simulink model "simlwrkuka_kinematics"  (R2014a)
settings: Solver=ode1  StartTime=0.0  StopTime=7  FixedStep=0.001  MaxStep=0.00001  RelTol=1e-3
values from neighbouring files (symbols this model uses):
  qi = [pi/2;0;0;pi/2;0;pi/2;pi/6]    [initial.m]
settings Model: Creator=Admin  LastModifiedBy=faezeh

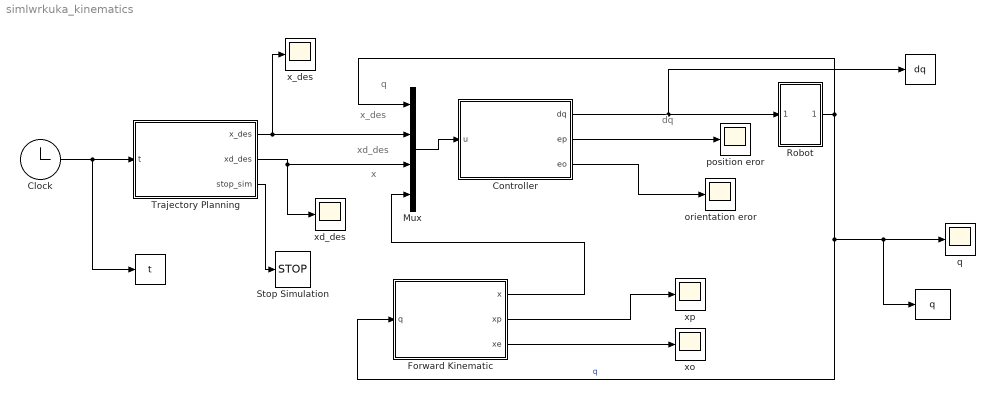
== system simlwrkuka_kinematics ==
  note: x
  note: dq
  note: q
  note: x_des
  note: xd_des
  " " : ToWorkspace  VariableName=q  SampleTime=-1
  "  " : ToWorkspace  VariableName=dq  SampleTime=-1
  " " : ToWorkspace  VariableName=t  SampleTime=-1
  Clock : Clock
  Controller : MATLAB Function  TreatAsAtomicUnit=on
  Forward Kinematic : MATLAB Function  TreatAsAtomicUnit=on
  Mux : Mux
  Robot : Subsystem
  Stop Simulation : Stop
  Trajectory Planning : MATLAB Function  TreatAsAtomicUnit=on
  orientation eror : Scope
  position eror : Scope
  q : Scope
      settings: SaveName=ScopeData2
  "x_des " : Scope
      settings: SaveName=ScopeData5
  "xd_des " : Scope
      settings: SaveName=ScopeData6
  xo : Scope
      settings: SaveName=ScopeData4
  xp : Scope
      settings: SaveName=ScopeData3
  wires:
  Clock/1 -> " "/1, Trajectory Planning/1(t)
  Trajectory Planning/3(stop_sim) -> Stop Simulation/1
  Mux/1 -> Controller/1(u)
  Controller/2(ep) -> position eror/1
  Trajectory Planning/1(x_des) -> "x_des "/1, Mux/2
  Trajectory Planning/2(xd_des) -> "xd_des "/1, Mux/3
  Controller/1(dq) -> "  "/1, Robot/1(In1)
  Robot/1(Out1) -> Forward Kinematic/1(q), " "/1, q/1, Mux/1  "q"
  Controller/3(eo) -> orientation eror/1
  Forward Kinematic/1(x) -> Mux/4
  Forward Kinematic/2(xp) -> xp/1
  Forward Kinematic/3(xe) -> xo/1

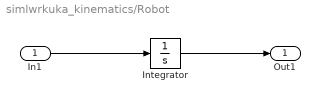
== system simlwrkuka_kinematics/Robot ==
  In1 : Inport
  Integrator : Integrator  InitialCondition=qi
  Out1 : Outport
  wires:
  Integrator/1 -> Out1/1
  In1/1 -> Integrator/1

== matlab function simlwrkuka_kinematics/Controller ==
  data: u input; dq output; ep output; eo output
function [dq,ep,eo] = command(u)
q1=u(1);q2=u(2);q3=u(3);q4=u(4);q5=u(5);q6=u(6);q7=u(7);
x_des=[u(8);u(9);u(10);u(11);u(12);u(13);u(14)];
xd_des=[u(15);u(16);u(17);u(18);u(19);u(20)];
x=[u(21);u(22);u(23);u(24);u(25);u(26);u(27)];
% J=[   (2*sin(q1)*sin(q2))/5 - (39*sin(q4)*(cos(q1)*sin(q3) + cos(q2)*cos(q3)*sin(q1)))/100 + (39*cos(q4)*sin(q1)*sin(q2))/100,                                                                                                                                                                                  -cos(q1)*((2*cos(q2))/5 + (39*cos(q2)*cos(q4))/100 + (39*cos(q3)*sin(q2)*sin(q4))/100),                                                     cos(q2)*((2*sin(q1)*sin(q2))/5 - (39*sin(q4)*(cos(q1)*sin(q3) + cos(q2)*cos(q3)*sin(q1)))/100 + (39*cos(q4)*sin(q1)*sin(q2))/100) - sin(q1)*sin(q2)*((2*cos(q2))/5 + (39*cos(q2)*cos(q4))/100 + (39*cos(q3)*sin(q2)*sin(q4))/100),                                                                 (cos(q1)*cos(q3) - cos(q2)*sin(q1)*sin(q3))*((39*cos(q2)*cos(q4))/100 + (39*cos(q3)*sin(q2)*sin(q4))/100) + sin(q2)*sin(q3)*((39*sin(q4)*(cos(q1)*sin(q3) + cos(q2)*cos(q3)*sin(q1)))/100 - (39*cos(q4)*sin(q1)*sin(q2))/100),                                                                         (sin(q4)*(cos(q1)*sin(q3) + cos(q2)*cos(q3)*sin(q1)) - cos(q4)*sin(q1)*sin(q2))*((39*cos(q2)*cos(q4))/100 + (39*cos(q3)*sin(q2)*sin(q4))/100) - ((39*sin(q4)*(cos(q1)*sin(q3) + cos(q2)*cos(q3)*sin(q1)))/100 - (39*cos(q4)*sin(q1)*sin(q2))/100)*(cos(q2)*cos(q4) + cos(q3)*sin(q2)*sin(q4)),                                                                                                                                             0,                                                                                                                                                                                                                                                 0
%  - (2*cos(q1)*sin(q2))/5 - (39*sin(q4)*(sin(q1)*sin(q3) - cos(q1)*cos(q2)*cos(q3)))/100 - (39*cos(q1)*cos(q4)*sin(q2))/100,                                                                                                                                                                                  -sin(q1)*((2*cos(q2))/5 + (39*cos(q2)*cos(q4))/100 + (39*cos(q3)*sin(q2)*sin(q4))/100),                                                     cos(q1)*sin(q2)*((2*cos(q2))/5 + (39*cos(q2)*cos(q4))/100 + (39*cos(q3)*sin(q2)*sin(q4))/100) - cos(q2)*((2*cos(q1)*sin(q2))/5 + (39*sin(q4)*(sin(q1)*sin(q3) - cos(q1)*cos(q2)*cos(q3)))/100 + (39*cos(q1)*cos(q4)*sin(q2))/100),                                                                 (cos(q3)*sin(q1) + cos(q1)*cos(q2)*sin(q3))*((39*cos(q2)*cos(q4))/100 + (39*cos(q3)*sin(q2)*sin(q4))/100) + sin(q2)*sin(q3)*((39*sin(q4)*(sin(q1)*sin(q3) - cos(q1)*cos(q2)*cos(q3)))/100 + (39*cos(q1)*cos(q4)*sin(q2))/100),                                                                         ((39*cos(q2)*cos(q4))/100 + (39*cos(q3)*sin(q2)*sin(q4))/100)*(sin(q4)*(sin(q1)*sin(q3) - cos(q1)*cos(q2)*cos(q3)) + cos(q1)*cos(q4)*sin(q2)) - (cos(q2)*cos(q4) + cos(q3)*sin(q2)*sin(q4))*((39*sin(q4)*(sin(q1)*sin(q3) - cos(q1)*cos(q2)*cos(q3)))/100 + (39*cos(q1)*cos(q4)*sin(q2))/100),                                                                                                                                             0,                                                                                                                                                                                                                                                 0
%                                                                                                                          0, - cos(q1)*((2*cos(q1)*sin(q2))/5 + (39*sin(q4)*(sin(q1)*sin(q3) - cos(q1)*cos(q2)*cos(q3)))/100 + (39*cos(q1)*cos(q4)*sin(q2))/100) - sin(q1)*((2*sin(q1)*sin(q2))/5 - (39*sin(q4)*(cos(q1)*sin(q3) + cos(q2)*cos(q3)*sin(q1)))/100 + (39*cos(q4)*sin(q1)*sin(q2))/100), cos(q1)*sin(q2)*((2*sin(q1)*sin(q2))/5 - (39*sin(q4)*(cos(q1)*sin(q3) + cos(q2)*cos(q3)*sin(q1)))/100 + (39*cos(q4)*sin(q1)*sin(q2))/100) - sin(q1)*sin(q2)*((2*cos(q1)*sin(q2))/5 + (39*sin(q4)*(sin(q1)*sin(q3) - cos(q1)*cos(q2)*cos(q3)))/100 + (39*cos(q1)*cos(q4)*sin(q2))/100), (cos(q1)*cos(q3) - cos(q2)*sin(q1)*sin(q3))*((39*sin(q4)*(sin(q1)*sin(q3) - cos(q1)*cos(q2)*cos(q3)))/100 + (39*cos(q1)*cos(q4)*sin(q2))/100) - ((39*sin(q4)*(cos(q1)*sin(q3) + cos(q2)*cos(q3)*sin(q1)))/100 - (39*cos(q4)*sin(q1)*sin(q2))/100)*(cos(q3)*sin(q1) + cos(q1)*cos(q2)*sin(q3)), (sin(q4)*(cos(q1)*sin(q3) + cos(q2)*cos(q3)*sin(q1)) - cos(q4)*sin(q1)*sin(q2))*((39*sin(q4)*(sin(q1)*sin(q3) - cos(q1)*cos(q2)*cos(q3)))/100 + (39*cos(q1)*cos(q4)*sin(q2))/100) - ((39*sin(q4)*(cos(q1)*sin(q3) + cos(q2)*cos(q3)*sin(q1)))/100 - (39*cos(q4)*sin(q1)*sin(q2))/100)*(sin(q4)*(sin(q1)*sin(q3) - cos(q1)*cos(q2)*cos(q3)) + cos(q1)*cos(q4)*sin(q2)),                                                                                                                                             0,                                                                                                                                                                                                                                                 0
%                                                                                                                          0,                                                                                                                                                                                                                                                                 sin(q1),                                                                                                                                                                                                                                                                      -cos(q1)*sin(q2),                                                                                                                                                                                                                                                   - cos(q3)*sin(q1) - cos(q1)*cos(q2)*sin(q3),                                                                                                                                                                                                                                                                                       - sin(q4)*(sin(q1)*sin(q3) - cos(q1)*cos(q2)*cos(q3)) - cos(q1)*cos(q4)*sin(q2), cos(q5)*(cos(q3)*sin(q1) + cos(q1)*cos(q2)*sin(q3)) - sin(q5)*(cos(q4)*(sin(q1)*sin(q3) - cos(q1)*cos(q2)*cos(q3)) - cos(q1)*sin(q2)*sin(q4)), sin(q6)*(cos(q5)*(cos(q4)*(sin(q1)*sin(q3) - cos(q1)*cos(q2)*cos(q3)) - cos(q1)*sin(q2)*sin(q4)) + sin(q5)*(cos(q3)*sin(q1) + cos(q1)*cos(q2)*sin(q3))) - cos(q6)*(sin(q4)*(sin(q1)*sin(q3) - cos(q1)*cos(q2)*cos(q3)) + cos(q1)*cos(q4)*sin(q2))
%                                                                                                                          0,                                                                                                                                                                                                                                                                -cos(q1),                                                                                                                                                                                                                                                                      -sin(q1)*sin(q2),                                                                                                                                                                                                                                                     cos(q1)*cos(q3) - cos(q2)*sin(q1)*sin(q3),                                                                                                                                                                                                                                                                                         sin(q4)*(cos(q1)*sin(q3) + cos(q2)*cos(q3)*sin(q1)) - cos(q4)*sin(q1)*sin(q2), sin(q5)*(cos(q4)*(cos(q1)*sin(q3) + cos(q2)*cos(q3)*sin(q1)) + sin(q1)*sin(q2)*sin(q4)) - cos(q5)*(cos(q1)*cos(q3) - cos(q2)*sin(q1)*sin(q3)), cos(q6)*(sin(q4)*(cos(q1)*sin(q3) + cos(q2)*cos(q3)*sin(q1)) - cos(q4)*sin(q1)*sin(q2)) - sin(q6)*(cos(q5)*(cos(q4)*(cos(q1)*sin(q3) + cos(q2)*cos(q3)*sin(q1)) + sin(q1)*sin(q2)*sin(q4)) + sin(q5)*(cos(q1)*cos(q3) - cos(q2)*sin(q1)*sin(q3)))
%                                                                                                                          1,                                                                                                                                                                                                                                                                       0,                                                                                                                                                                                                                                                                               cos(q2),                                                                                                                                                                                                                                                                              -sin(q2)*sin(q3),                                                                                                                                                                                                                                                                                                                             cos(q2)*cos(q4) + cos(q3)*sin(q2)*sin(q4),                                                                 cos(q5)*sin(q2)*sin(q3) - sin(q5)*(cos(q2)*sin(q4) - cos(q3)*cos(q4)*sin(q2)),                                                                                                     sin(q6)*(cos(q5)*(cos(q2)*sin(q4) - cos(q3)*cos(q4)*sin(q2)) + sin(q2)*sin(q3)*sin(q5)) + cos(q6)*(cos(q2)*cos(q4) + cos(q3)*sin(q2)*sin(q4))];
% T7=[ sin(q7)*(sin(q5)*(cos(q4)*(sin(q1)*sin(q3) - cos(q1)*cos(q2)*cos(q3)) - cos(q1)*sin(q2)*sin(q4)) - cos(q5)*(cos(q3)*sin(q1) + cos(q1)*cos(q2)*sin(q3))) - cos(q7)*(sin(q6)*(sin(q4)*(sin(q1)*sin(q3) - cos(q1)*cos(q2)*cos(q3)) + cos(q1)*cos(q4)*sin(q2)) + cos(q6)*(cos(q5)*(cos(q4)*(sin(q1)*sin(q3) - cos(q1)*cos(q2)*cos(q3)) - cos(q1)*sin(q2)*sin(q4)) + sin(q5)*(cos(q3)*sin(q1) + cos(q1)*cos(q2)*sin(q3)))),   sin(q7)*(sin(q6)*(sin(q4)*(sin(q1)*sin(q3) - cos(q1)*cos(q2)*cos(q3)) + cos(q1)*cos(q4)*sin(q2)) + cos(q6)*(cos(q5)*(cos(q4)*(sin(q1)*sin(q3) - cos(q1)*cos(q2)*cos(q3)) - cos(q1)*sin(q2)*sin(q4)) + sin(q5)*(cos(q3)*sin(q1) + cos(q1)*cos(q2)*sin(q3)))) + cos(q7)*(sin(q5)*(cos(q4)*(sin(q1)*sin(q3) - cos(q1)*cos(q2)*cos(q3)) - cos(q1)*sin(q2)*sin(q4)) - cos(q5)*(cos(q3)*sin(q1) + cos(q1)*cos(q2)*sin(q3))), sin(q6)*(cos(q5)*(cos(q4)*(sin(q1)*sin(q3) - cos(q1)*cos(q2)*cos(q3)) - cos(q1)*sin(q2)*sin(q4)) + sin(q5)*(cos(q3)*sin(q1) + cos(q1)*cos(q2)*sin(q3))) - cos(q6)*(sin(q4)*(sin(q1)*sin(q3) - cos(q1)*cos(q2)*cos(q3)) + cos(q1)*cos(q4)*sin(q2)), - (2*cos(q1)*sin(q2))/5 - (39*sin(q4)*(sin(q1)*sin(q3) - cos(q1)*cos(q2)*cos(q3)))/100 - (39*cos(q1)*cos(q4)*sin(q2))/100
%  cos(q7)*(sin(q6)*(sin(q4)*(cos(q1)*sin(q3) + cos(q2)*cos(q3)*sin(q1)) - cos(q4)*sin(q1)*sin(q2)) + cos(q6)*(cos(q5)*(cos(q4)*(cos(q1)*sin(q3) + cos(q2)*cos(q3)*sin(q1)) + sin(q1)*sin(q2)*sin(q4)) + sin(q5)*(cos(q1)*cos(q3) - cos(q2)*sin(q1)*sin(q3)))) - sin(q7)*(sin(q5)*(cos(q4)*(cos(q1)*sin(q3) + cos(q2)*cos(q3)*sin(q1)) + sin(q1)*sin(q2)*sin(q4)) - cos(q5)*(cos(q1)*cos(q3) - cos(q2)*sin(q1)*sin(q3))), - sin(q7)*(sin(q6)*(sin(q4)*(cos(q1)*sin(q3) + cos(q2)*cos(q3)*sin(q1)) - cos(q4)*sin(q1)*sin(q2)) + cos(q6)*(cos(q5)*(cos(q4)*(cos(q1)*sin(q3) + cos(q2)*cos(q3)*sin(q1)) + sin(q1)*sin(q2)*sin(q4)) + sin(q5)*(cos(q1)*cos(q3) - cos(q2)*sin(q1)*sin(q3)))) - cos(q7)*(sin(q5)*(cos(q4)*(cos(q1)*sin(q3) + cos(q2)*cos(q3)*sin(q1)) + sin(q1)*sin(q2)*sin(q4)) - cos(q5)*(cos(q1)*cos(q3) - cos(q2)*sin(q1)*sin(q3))), cos(q6)*(sin(q4)*(cos(q1)*sin(q3) + cos(q2)*cos(q3)*sin(q1)) - cos(q4)*sin(q1)*sin(q2)) - sin(q6)*(cos(q5)*(cos(q4)*(cos(q1)*sin(q3) + cos(q2)*cos(q3)*sin(q1)) + sin(q1)*sin(q2)*sin(q4)) + sin(q5)*(cos(q1)*cos(q3) - cos(q2)*sin(q1)*sin(q3))),   (39*sin(q4)*(cos(q1)*sin(q3) + cos(q2)*cos(q3)*sin(q1)))/100 - (2*sin(q1)*sin(q2))/5 - (39*cos(q4)*sin(q1)*sin(q2))/100
%                                                                                                                                                                      sin(q7)*(sin(q5)*(cos(q2)*sin(q4) - cos(q3)*cos(q4)*sin(q2)) - cos(q5)*sin(q2)*sin(q3)) - cos(q7)*(cos(q6)*(cos(q5)*(cos(q2)*sin(q4) - cos(q3)*cos(q4)*sin(q2)) + sin(q2)*sin(q3)*sin(q5)) - sin(q6)*(cos(q2)*cos(q4) + cos(q3)*sin(q2)*sin(q4))),                                                                                                                                                                       cos(q7)*(sin(q5)*(cos(q2)*sin(q4) - cos(q3)*cos(q4)*sin(q2)) - cos(q5)*sin(q2)*sin(q3)) + sin(q7)*(cos(q6)*(cos(q5)*(cos(q2)*sin(q4) - cos(q3)*cos(q4)*sin(q2)) + sin(q2)*sin(q3)*sin(q5)) - sin(q6)*(cos(q2)*cos(q4) + cos(q3)*sin(q2)*sin(q4))),                                                                                                     sin(q6)*(cos(q5)*(cos(q2)*sin(q4) - cos(q3)*cos(q4)*sin(q2)) + sin(q2)*sin(q3)*sin(q5)) + cos(q6)*(cos(q2)*cos(q4) + cos(q3)*sin(q2)*sin(q4)),                                               (2*cos(q2))/5 + (39*cos(q2)*cos(q4))/100 + (39*cos(q3)*sin(q2)*sin(q4))/100
%                                                                                                                                                                                                                                                                                                                                                                                                                      0,                                                                                                                                                                                                                                                                                                                                                                                                                       0,                                                                                                                                                                                                                                                 0,                                                                                                                         1];
[J,Te]=jacobin(q1,q2,q3,q4,q5,q6,q7);
Re=Te(1:3,1:3);
kp=15;
kpo=4;
eps=x(5:7);
eta=x(4);
eta_des=x_des(4);
eps_des=x_des(5:7);
S_eps=[0 -eps(3) eps(2); eps(3) 0 -eps(1);-eps(2) eps(1) 0];
eps_de=(eta*eps_des-eta_des*eps-S_eps*eps_des);
xd_com_o=xd_des(4:6)+kpo*Re*eps_de;
xd_com_p=xd_des(1:3)+kp*(x_des(1:3)-x(1:3));
Xd_com=[xd_com_p;xd_com_o];
dq=pinv(J)*Xd_com;
ep=x_des(1:3)-x(1:3);
eo=x_des(4:6)-x(4:6);

== matlab function simlwrkuka_kinematics/Trajectory Planning ==
  data: t input; x_des output; xd_des output; stop_sim output
function [x_des,xd_des,stop_sim] = TRJ(t)
%linear trajectory
   xf=[0.085;-0.085;0.597]; %Linear Trajectory Final Point
   xi=[0;-0.39;0.61]; %Linear Trajectory Initial Point
   L=norm(xf-xi);
   v_max=0.05; %v_max~L/7
   T=7;
   a_max=v_max^2/(T*v_max-L);
   stop_sim=0;
   sig=0;
   sigd=0;
%    sigdd=0;

   Ts=v_max/a_max;
   if t<=Ts
   sig=a_max*t^2/2;
   sigd=a_max*t;
%    sigdd=a_max;
   elseif t>Ts && t<=(T-Ts)
   sig=v_max*t-(v_max)^2/(2*a_max);
   sigd=v_max;
%    sigdd=0;
   elseif t>(T-Ts) && t<=T
   sig=-a_max*(t-T)^2/2+v_max*T-(v_max)^2/a_max;
   sigd=-a_max*(t-T);
%    sigdd=-a_max;
   else
       stop_sim=1;
   end
   R_des=[-0.866 -0.5 0;0.5 -0.866 0;0 0 1];
%    f_des=atan2(R(2,1),R(1,1));
%    t_des=atan2(-R(3,1),sqrt(R(3,2)^2+R(3,3)^2));
%    s_des=atan2(R(3,2),R(3,3)); 
%    RPY_des=[s_des;t_des;f_des]; %RPY Representation
%    t_des=2.6180;f_des=0;s_des=0; 
%    euler_des=[t_des;f_des;s_des]; %Euler Representation
   eta_des=0.5*sqrt(R_des(1,1)+R_des(2,2)+R_des(3,3)+1);
   e_des=0.5*[sign(R_des(3,2)-R_des(2,3))*sqrt((R_des(1,1)-R_des(2,2)-R_des(3,3)+1));
              sign(R_des(1,3)-R_des(3,1))*sqrt((R_des(2,2)-R_des(3,3)-R_des(1,1)+1));
              sign(R_des(2,1)-R_des(1,2))*sqrt((R_des(3,3)-R_des(1,1)-R_des(2,2)+1))];
   Q_des=[eta_des;e_des]; %Unit Quaternion Representation
   x_des=[xi+sig*(xf-xi)/L;Q_des]; %7
   xd_des=[(xf-xi)/L*sigd;0;0;0]; %6
%  xdd_des=(xf-xi)/L*sigdd;

== matlab function simlwrkuka_kinematics/Forward Kinematic ==
  data: q input; x output; xp output; xe output
function [x,xp,xe]  = command(q)
q1=q(1);q2=q(2);q3=q(3);q4=q(4);q5=q(5);q6=q(6);q7=q(7);
[~,Te]=jacobin(q1,q2,q3,q4,q5,q6,q7);
p=Te(1:3,4);
R7=Te(1:3,1:3);
% f=atan2(R7(2,1),R7(1,1));
% t=atan2(-R7(3,1),sqrt(R77(3,2)^2+R7(3,3)^2));
% s=atan2(R7(3,2),R7(3,3)); 
% RPY=[s;t;f]; %R7PY R7epR7esentation
% f=atan2(R7(2,1),R7(1,1));
% t=atan2(-R7(3,1),sqrt(R7(3,2)^2+R7(3,3)^2));
% s=atan2(R7(3,2),R7(3,3));
% euler=[f;t;s];
% x=[p;RPY];
eta=0.5*sqrt(R7(1,1)+R7(2,2)+R7(3,3)+1);
e=0.5*[sign(R7(3,2)-R7(2,3))*sqrt((R7(1,1)-R7(2,2)-R7(3,3)+1));
              sign(R7(1,3)-R7(3,1))*sqrt((R7(2,2)-R7(3,3)-R7(1,1)+1));
              sign(R7(2,1)-R7(1,2))*sqrt((R7(3,3)-R7(1,1)-R7(2,2)+1))];
Q=[eta;e];
x=[p;Q];
xp=x(1:3);
xe=x(4:6);
